simulink model "PMSM_FOC_Average_Inveter"  (R2020b)
settings: Solver=FixedStepAuto  StartTime=0.0  StopTime=10  FixedStep=Fixed_Step_Size  RelTol=1e-3
model workspace (MAT data in the model file):
  wc = Simulink.Parameter
  wc.DataType = 'auto'
  wc.Dimensions = [0 0]
values from neighbouring files (symbols this model uses):
  Angle = 1.0    [Motor_Control_Data.sldd]
  Cosine_table = 1.0 0.99999529 0.99999058 0.99998587 0.99998116 0.99996704 0.99995291 0.99993885 0.99992472 0.99990118 0.99987763 0.99985409 0.9998306 0.99979764 0.99976468 0.99973178 0.99969882 0.99965644 0.99961412 0.99957174 0.99952942 0.99947762 0.99942589 0.99937415 0.99932235 0.9992612 0.99920005 0.99913889 0.99907768 0.99900717 0.99893659 0.99886602 0.99879545 0.99871546 0.99863547 0.99855554 0.99847555 0.    [Motor_Control_Data.sldd]
  Fixed_Step_Size = 1.0E-5    [Motor_Control_Data.sldd]
  Flux = 0.1125    [Motor_Control_Data.sldd]
  ID_Ki = 48.0    [Motor_Control_Data.sldd]
  ID_Kp = 0.84    [Motor_Control_Data.sldd]
  IQ_Ki = 48.0    [Motor_Control_Data.sldd]
  IQ_Kp = 1.869    [Motor_Control_Data.sldd]
  Ld = 0.00014    [Motor_Control_Data.sldd]
  Lq = 0.0003115    [Motor_Control_Data.sldd]
  MTPA_Te_Min = 0.0    [Motor_Control_Data.sldd]
  Pole_Pairs = 4.0    [Motor_Control_Data.sldd]
  PWM_Frequency = 10000.0    [Motor_Control_Data.sldd]
  Sine_table = 0.0 0.0015339879 0.0030679768 0.0046019657 0.0061359555 0.0076698866 0.0092038177 0.010737749 0.012271681 0.013805497 0.015339312 0.016873131 0.018406944 0.019940587 0.021474229 0.023007872 0.024541514 0.026074925 0.027608337 0.029141748 0.03067516 0.032208283 0.033741407 0.035274528 0.036807653 0.038340431 0.039873205 0.04140598 0.042938754 0.04447113 0.046003502 0.047535874 0.049068246 0.0506001    [Motor_Control_Data.sldd]
  Speed_Ki = 10.809    [Motor_Control_Data.sldd]
  Speed_Kp = 0.08    [Motor_Control_Data.sldd]
  Speed_PI_OutputMax = 700.0    [Motor_Control_Data.sldd]
  Speed_PI_OutputMin = -700.0    [Motor_Control_Data.sldd]
  TorqueMode = 0.0    [Motor_Control_Data.sldd]
undefined symbols (not defined in the file or in its folder): Angle_offset, DiscIntNeverNeededParam, FluxWeak_Enable, FluxWeak_Idref_max, FluxWeak_Idref_min, FluxWeak_Ki, FluxWeak_Kp, inverter, MTPA_id_table, MTPA_iq_table, MTPA_Te_Max, Over_modulation, sigbuilder_block, SVPWM
libraries: simulink x7, pid_lib x1, mcbplantlib x1, autolibpmsminterior x1
(part 1 of 2)
settings Model: DataDictionary=Motor_Control_Data.sldd  Creator=jt  LastModifiedBy=Administrator
settings DataIOCC: LimitDataPoints=on  SaveFormat=Array  ReturnWorkspaceOutputs=off
settings OptimizationCC: DefaultParameterBehavior=Inlined  UseDivisionForNetSlopeComputation=on  GainParamInheritBuiltInType=on  UseFloatMulNetSlope=on  InlineInvariantSignals=on  PassReuseOutputArgsAs=Individual arguments  ZeroExternalMemoryAtStartup=off  NoFixptDivByZeroProtection=on  EfficientFloat2IntCast=on  LifeSpan=1  OptimizeBlockOrder=speed  DifferentSizesBufferReuse=on  EfficientTunableParamExpr=on
settings DebuggingCC: AlgebraicLoopMsg=none  MaxConsecutiveZCsMsg=none  SolverPrmCheckMsg=warning  ParameterTunabilityLossMsg=error  AllowSymbolicDim=off  SFUnexpectedBacktrackingDiag=warning  SFNoUnconditionalDefaultTransitionDiag=warning  SFExecutionAtInitializationDiag=none  ArithmeticOperatorsInVariantConditions=warning
settings HardwareCC: ProdBitPerPointer=32  ProdBitPerSizeT=32  ProdBitPerPtrDiffT=32  ProdLargestAtomicInteger=Long  ProdLargestAtomicFloat=Double  ProdEndianess=BigEndian  ProdWordSize=32  ProdLongLongMode=on  ProdHWDeviceType=Freescale->32-bit PowerPC
settings ModelReferenceCC: PropagateSignalLabelsOutOfModel=off
settings SFSimCC: SimUseLocalCustomCode=off  SimParseCustomCode=off  MATLABDynamicMemAlloc=off  CustomCodeUndefinedFunction=UseInterfaceOnly
settings RTWCC: Description=Embedded Coder  SystemTargetFile=ert.tlc  GenCodeOnly=on  TemplateMakefile=ert_default_tmf  GenerateReport=on  RTWUseLocalCustomCode=off  IncludeHyperlinkInReport=on  LaunchReport=on  GenerateTraceInfo=on  GenerateTraceReport=on  GenerateTraceReportSl=on  GenerateTraceReportSf=on  GenerateTraceReportEml=on  GenerateCodeMetricsReport=on
settings CodeAppCC: ForceParamTrailComments=on  IgnoreCustomStorageClasses=off  OperatorAnnotations=on  SimulinkDataObjDesc=on  SFDataObjDesc=on  CustomSymbolStrGlobalVar=rt$N$M  CustomSymbolStrType=$N$M  CustomSymbolStrFcn=$N$M$F  CustomSymbolStrMacro=$N$M  InsertBlockDesc=on
settings ERTTargetCC: GenerateSampleERTMain=on  IncludeMdlTerminateFcn=off  CombineSignalStateStructs=on  SupportAbsoluteTime=off  SupportNonFinite=off  SupportComplex=off  SupportNonInlinedSFcns=on  InlinedParameterPlacement=NonHierarchical  ERTCustomFileTemplate=example_file_process.tlc
settings ConfigComp: CovMetricSettings=dw  CovSaveCumulativeToWorkspaceVar=on  CovSaveSingleToWorkspaceVar=on  CovExternalEMLEnable=off  CovSFcnEnable=off  PSAutoStubLUT=on  DVTestSuiteOptimization=Auto  DVDetectDeadLogic=on  DVDetectActiveLogic=on  DVDetectOutOfBounds=on  DVSaveReport=on  DVDisplayReport=off
settings SimscapeCC: SimscapeNormalizeSystem=off

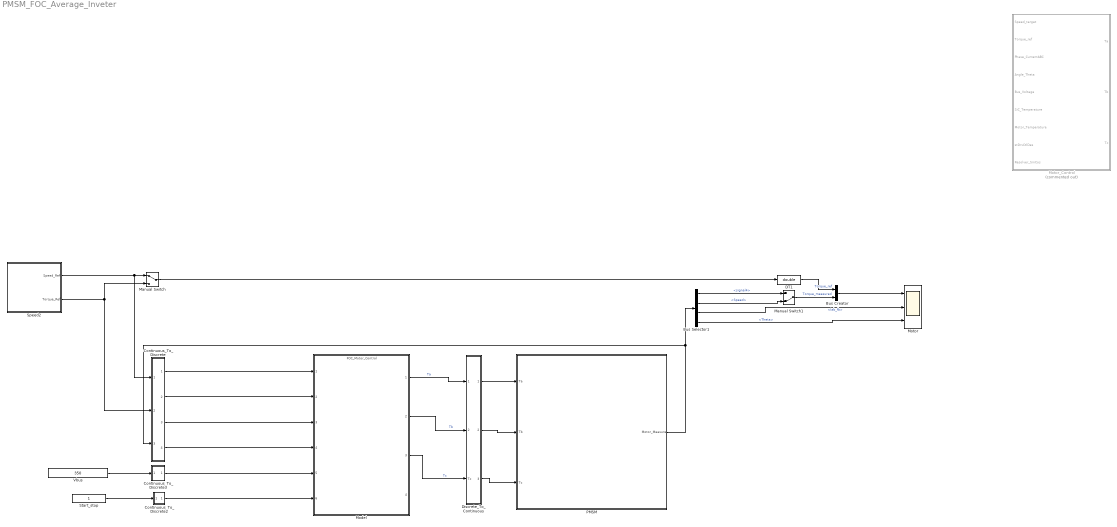
== system PMSM_FOC_Average_Inveter ==
  Bus Creator : BusCreator  Inputs=2
  Bus Selector1 : BusSelector  OutputSignals=signal4,Speed,Iab_fb,Theta
  Continuous_To_Discrete : Subsystem
      mask Display: fprintf('C/D')
  Continuous_To_Discrete2 : Subsystem
      mask Display: fprintf('C/D')
  Continuous_To_Discrete3 : Subsystem
      mask Display: fprintf('C/D')
  DT1 : DataTypeConversion  OutDataTypeStr=double
  Discrete_To_Continuous : Subsystem  Description=""
      mask Display: fprintf('D/C')
  Manual Switch : ManualSwitch
  Manual Switch1 : ManualSwitch  CurrentSetting=0
  Model : ModelReference  ModelNameDialog=FOC_Motor_Control.slx  SimulationMode=Normal  CodeInterface=Top model  ModelReferenceVersion=1.40
  Motor : Scope  NumInputPorts=3
  Motor_Control : Subsystem  Commented=on  TreatAsAtomicUnit=on
  PMSM : Subsystem
      mask Display: image('$imagefile'); % Use "Edit Image" on toolstrip to change.
  Speed2 : Subsystem  Tag=STV Subsys  LoadFcn=sigbuilder_block('load');  StartFcn=sigbuilder_block('start');  StopFcn=sigbuilder_block('stop');  ClipboardFcn=sigbuilder_block('clipboard');  mask(Sigbuilder block){tuvar=[0:10]}
      mask help: Simulink:masks:SigbuilderBlock_MD
      mask init:
      | if ~strcmp(get_param(bdroot(gcbh),'SimulationStatus'),'stopped') tuvar = sigbuilder_block('maskInit'); end
      settings: CopyFcn=sigbuilder_block('copy');  DeleteFcn=sigbuilder_block('delete');  ModelCloseFcn=sigbuilder_block('modelClose');  PreSaveFcn=sigbuilder_block('preSave');  PauseFcn=sigbuilder_block('pause');  ContinueFcn=sigbuilder_block('continue');  NameChangeFcn=sigbuilder_block('namechange');  OpenFcn=sigbuilder_block('open',[48.5 0 906 449 ]);  CloseFcn=sigbuilder_block('close');
      mask Display: plot(0, 0, 100, 100,[2, 2, 32, 32, 2], [68, 8, 8, 68, 68],[32, 2], [38, 38], [32, 19, 2],[53, 60, 44], [32, 17, 17, 2],[16, 16, 31, 31]);txt = getActiveGroup(gcbh);text(2, 100, txt,'verticalAlignment', 'top');
  Start_stop : Constant  OutDataTypeStr=uint8
  Vbus : Constant  Value=350  OutDataTypeStr=single
  wires:
  Discrete_To_Continuous/1(T1) -> PMSM/1(Ta)
  Discrete_To_Continuous/2(T2) -> PMSM/2(Tb)
  Discrete_To_Continuous/3(T3) -> PMSM/3(Tc)
  PMSM/1(Motor_Measure) -> Bus Selector1/1, Continuous_To_Discrete/3(Motor_Measurements)
  Continuous_To_Discrete/4(Theta) -> Model/4
  Model/1 -> Discrete_To_Continuous/1(Ta)  "Ta"
  Model/2 -> Discrete_To_Continuous/2(Tb)  "Tb"
  Model/3 -> Discrete_To_Continuous/3(Tc)  "Tc"
  Bus Creator/1 -> Motor/1
  Bus Selector1/3 -> Motor/2  "<Iab_fb>"
  Speed2/1(Speed_Ref) -> Continuous_To_Discrete/1(Speed_Command), Manual Switch/1
  Continuous_To_Discrete/3(Phase_CurrentABC) -> Model/3
  Bus Selector1/4 -> Motor/3  "<Theta>"
  Start_stop/1 -> Continuous_To_Discrete2/1(Start_stop)
  Speed2/2(Torque_Ref) -> Continuous_To_Discrete/2(Torque_command), Manual Switch/2
  Manual Switch/1 -> DT1/1
  Bus Selector1/1 -> Manual Switch1/1  "<signal4>"
  Bus Selector1/2 -> Manual Switch1/2  "<Speed>"
  Manual Switch1/1 -> Bus Creator/2  "Torque_measured"
  Continuous_To_Discrete2/1(Enable_Disable) -> Model/6
  Continuous_To_Discrete/2(Torque_ref) -> Model/2
  DT1/1 -> Bus Creator/1  "Torque_ref"
  Continuous_To_Discrete/1(Speed_target) -> Model/1
  Vbus/1 -> Continuous_To_Discrete3/1(Bus_Voltage)
  Continuous_To_Discrete3/1(Vbus) -> Model/5

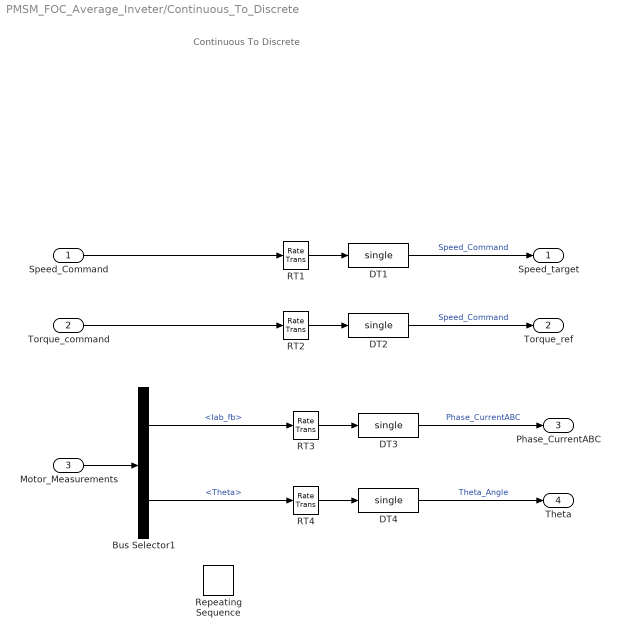
== system PMSM_FOC_Average_Inveter/Continuous_To_Discrete ==
  note: Continuous To Discrete
  Speed_Command : Inport
  Torque_command : Inport  Port=2
  Motor_Measurements : Inport  Port=3
  Bus Selector1 : BusSelector  OutputSignals=Iab_fb,Theta
  DT{1..4} (4 alike) : DataTypeConversion  OutDataTypeStr=single
  RT{1..4} (4 alike) : RateTransition  Integrity=off
  Repeating Sequence : simulink/Sources/Repeating Sequence  rep_seq_t=[0 0.1]  rep_seq_y=[0 6.28]
  Speed_target : Outport
  Torque_ref : Outport  Port=2
  Phase_CurrentABC : Outport  Port=3  PortDimensions=3
  Theta : Outport  Port=4
  wires:
  DT1/1 -> Speed_target/1  "Speed_Command"
  RT1/1 -> DT1/1
  RT3/1 -> DT3/1
  Motor_Measurements/1 -> Bus Selector1/1
  Speed_Command/1 -> RT1/1
  RT4/1 -> DT4/1
  DT4/1 -> Theta/1  "Theta_Angle"
  Bus Selector1/1 -> RT3/1  "<Iab_fb>"
  DT3/1 -> Phase_CurrentABC/1  "Phase_CurrentABC"
  Bus Selector1/2 -> RT4/1  "<Theta>"
  Torque_command/1 -> RT2/1
  RT2/1 -> DT2/1
  DT2/1 -> Torque_ref/1  "Speed_Command"

== system PMSM_FOC_Average_Inveter/Continuous_To_Discrete2 ==
  note: Continuous To Discrete
  Start_stop : Inport
  DT1 : DataTypeConversion  OutDataTypeStr=uint8
  RT1 : RateTransition  Integrity=off
  Enable_Disable : Outport
  wires:
  DT1/1 -> Enable_Disable/1
  RT1/1 -> DT1/1
  Start_stop/1 -> RT1/1

== system PMSM_FOC_Average_Inveter/Continuous_To_Discrete3 ==
  note: Continuous To Discrete
  Bus_Voltage : Inport
  DT2 : DataTypeConversion  OutDataTypeStr=single
  RT2 : RateTransition  Integrity=off
  Vbus : Outport
  wires:
  Bus_Voltage/1 -> RT2/1
  RT2/1 -> DT2/1
  DT2/1 -> Vbus/1

== system PMSM_FOC_Average_Inveter/Discrete_To_Continuous ==
  note: Discrete To Continuous
  Ta : Inport
  Tb : Inport  Port=2
  Tc : Inport  Port=3
  DT : DataTypeConversion
  DT1 : DataTypeConversion
  DT2 : DataTypeConversion
  RT : RateTransition  Integrity=off
  RT1 : RateTransition  Integrity=off
  RT2 : RateTransition  Integrity=off
  T1 : Outport
  T2 : Outport  Port=2
  T3 : Outport  Port=3
  wires:
  DT/1 -> RT/1
  Ta/1 -> DT/1  "Tabc"
  DT1/1 -> RT1/1
  Tb/1 -> DT1/1  "Tabc"
  DT2/1 -> RT2/1
  Tc/1 -> DT2/1  "Tabc"
  RT/1 -> T1/1  "Tabc"
  RT1/1 -> T2/1  "Tabc"
  RT2/1 -> T3/1  "Tabc"

== system PMSM_FOC_Average_Inveter/Motor_Control ==
  Speed_target : Inport
  Torque_ref : Inport  Port=2  OutMin=0  OutMax=2*pi
  Phase_CurrentABC : Inport  Port=3  PortDimensions=3
  Angle_Theta : Inport  Port=4  OutMin=0  OutMax=2*pi
  Bus_Voltage : Inport  Port=5
  SiC_Temperature : Inport  Port=6
  Motor_Temperature : Inport  Port=7
  stDrvCtlDes : Inport  Port=8
  Resolver_SinCos : Inport  Port=9  OutMin=0  OutMax=2*pi
  Motor_Control_Function : Subsystem
  Ta : Outport
  Tb : Outport  Port=2
  Tc : Outport  Port=3
  wires:
  Motor_Control_Function/2(Tb) -> Tb/1
  Motor_Control_Function/3(Tc) -> Tc/1
  Motor_Control_Function/1(Ta) -> Ta/1
  Speed_target/1 -> Motor_Control_Function/1(Speed_target)  "Speed_target"
  Phase_CurrentABC/1 -> Motor_Control_Function/2(Phase_CurrentABC)  "Phase_CurrentABC"
  Angle_Theta/1 -> Motor_Control_Function/3(Angle_Theta)  "Angle_Theta"
  Resolver_SinCos/1 -> Motor_Control_Function/4(Resolver_SinCos)  "Resolver_signal"
  stDrvCtlDes/1 -> Motor_Control_Function/16(stDrvCtlDes)
  Bus_Voltage/1 -> Motor_Control_Function/5(Bus_voltage)
  SiC_Temperature/1 -> Motor_Control_Function/6(SiC_Temperature)
  Motor_Temperature/1 -> Motor_Control_Function/7(Motor_Temperature)
  Torque_ref/1 -> Motor_Control_Function/22(Torque_ref)

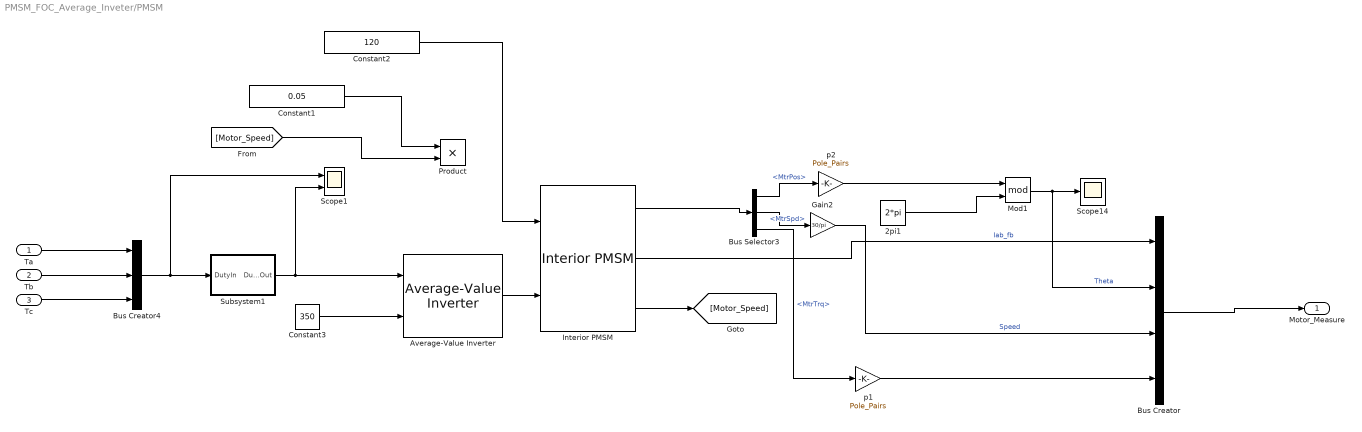
== system PMSM_FOC_Average_Inveter/PMSM ==
  Ta : Inport
  Tb : Inport  Port=2
  Tc : Inport  Port=3
  2pi1 : Constant  Value=2*pi
  Average-Value Inverter : mcbplantlib/Average-Value Inverter
  Bus Creator : BusCreator  Inputs=4
  Bus Creator4 : BusCreator  Inputs=3
  Bus Selector3 : BusSelector  OutputSignals=MtrPos,MtrSpd,MtrTrq
  Constant1 : Constant  Value=0.05
  Constant2 : Constant  Value=120
  Constant3 : Constant  Value=350
  Gain2 : Gain  Gain=30/pi  OutDataTypeStr=Inherit: Same as input  ParamDataTypeStr=Inherit: Same as input
  Interior PMSM : autolibpmsminterior/Interior PMSM  port_config=Torque  sim_type=Discrete  Ts=Fixed_Step_Size  P=Pole_Pairs  Rs=R  Ldq=[Ld Lq]  KConstText=Permanent flux linkage constant (lambda_pm):  lambda_pm=Flux  Ke=159.9771  mechanical=[0.002,0,0]  idq0=[0 0]  theta_init=0  omega_init=0  KConst=Flux  lambda_pm_calc=Flux  Kt=0.07  RefBlkName='autolibpmsminterior/Interior PMSM'  aMode=5
      settings: SourceProductBaseCode=PW,MT,UV,VE,VP
  Mod1 : Math  Operator=mod  SaturateOnIntegerOverflow=on
  Product : Product
  Scope1 : Scope  NumInputPorts=2
  Scope14 : Scope
  Subsystem1 : Subsystem
  p1 : Gain  Gain=Pole_Pairs  OutDataTypeStr=Inherit: Same as input  ParamDataTypeStr=Inherit: Same as input
  p2 : Gain  Gain=Pole_Pairs  OutDataTypeStr=Inherit: Same as input  ParamDataTypeStr=Inherit: Same as input
  Motor_Measure : Outport
  wires:
  Mod1/1 -> Bus Creator/2, Scope14/1  "Theta"
  Bus Creator/1 -> Motor_Measure/1
  Tc/1 -> Bus Creator4/3
  Interior PMSM/1 -> Bus Selector3/1
  Average-Value Inverter/1 -> Interior PMSM/2
  Subsystem1/1(DutyOut) -> Scope1/2, Average-Value Inverter/1
  Constant3/1 -> Average-Value Inverter/2
  Interior PMSM/2 -> Bus Creator/1  "Iab_fb"
  Bus Creator4/1 -> Subsystem1/1(DutyIn), Scope1/1
  Bus Selector3/2 -> Gain2/1  "<MtrSpd>"
  Bus Selector3/1 -> p2/1  "<MtrPos>"
  p2/1 -> Mod1/1
  2pi1/1 -> Mod1/2
  Gain2/1 -> Bus Creator/3  "Speed"
  Ta/1 -> Bus Creator4/1
  Tb/1 -> Bus Creator4/2
  Interior PMSM/3 -> [Motor_Speed]
  Bus Selector3/3 -> p1/1  "<MtrTrq>"
  p1/1 -> Bus Creator/4
  [Motor_Speed] -> Product/2
  Constant1/1 -> Product/1
  Constant2/1 -> Interior PMSM/1

== system PMSM_FOC_Average_Inveter/Speed2 ==
  Demux : Demux  Tag=STV Demux  Outputs=2
      settings: DisplayOption=none
  FromWs : FromWorkspace  Tag=STV FromWs  VariableName=tuvar
      SigBuilderData=|
      | common.afterFinalStr = 'Extrapolate'
      | common.sampleTime = 0
      | dataSet.timeRange = [0 10]
      | dataSet.name = 'Target Speed'
      | sbobj.Groups.Name = 'Target Speed'
      | sbobj.Groups.Signals(1).Name = 'Speed_Ref'
      | sbobj.Groups.Signals(1).XData = [0 4.51 10]
      | sbobj.Groups.Signals(1).YData = [2000 2000 2000]
      | sbobj.Groups.Signals(2).Name = 'Torque_Ref'
      | sbobj.Groups.Signals(2).XData = [0 1.26 1.26 2.9 5.44 5.44 7.94 10]
      | sbobj.Groups.Signals(2).YData = [170 170 169.5 170.5 170.5 170 170 170]
  Speed_Ref : Outport  Tag=STV Outport
  Torque_Ref : Outport  Tag=STV Outport  Port=2
  wires:
  FromWs/1 -> Demux/1
  Demux/1 -> Speed_Ref/1
  Demux/2 -> Torque_Ref/1

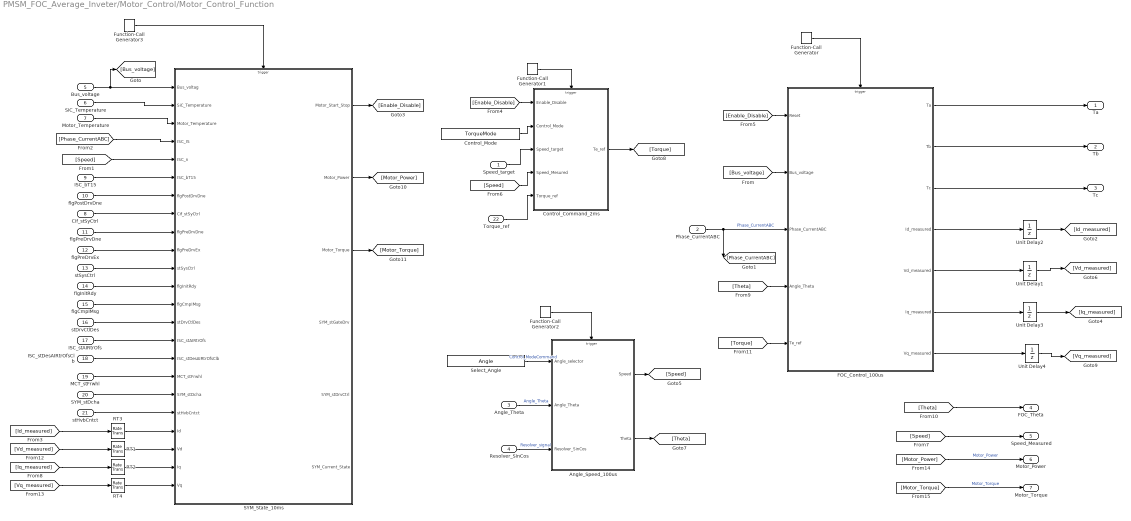
== system PMSM_FOC_Average_Inveter/Motor_Control/Motor_Control_Function ==
  Speed_target : Inport
  Phase_CurrentABC : Inport  Port=2  PortDimensions=3
  Angle_Theta : Inport  Port=3  OutMin=0  OutMax=2*pi
  Resolver_SinCos : Inport  Port=4  OutMin=0  OutMax=2*pi
  Bus_voltage : Inport  Port=5
  SiC_Temperature : Inport  Port=6
  Motor_Temperature : Inport  Port=7
  Cif_stSyCtrl : Inport  Port=8
  ISC_bT15 : Inport  Port=9
  flgPostDrvDne : Inport  Port=10
  flgPreDrvDne : Inport  Port=11
  flgPreDrvEx : Inport  Port=12
  stSysCtrl : Inport  Port=13
  flgInitRdy : Inport  Port=14
  flgCmpIMsg : Inport  Port=15
  stDrvCtlDes : Inport  Port=16
  ISC_stAIRtrOfs : Inport  Port=17
  "ISC_stDesAIRtrOfsClb " : Inport  Port=18
  MCT_stFrwhl : Inport  Port=19
  SYM_stDcha : Inport  Port=20
  stHvbCntct : Inport  Port=21
  Torque_ref : Inport  Port=22  OutMin=0  OutMax=2*pi
  Angle_Speed_100us : Subsystem
      settings: RTWSystemCode=Nonreusable function  RTWFcnNameOpts=Use subsystem name  RTWFileNameOpts=Use subsystem name
  Control_Command_2ms : Subsystem  TreatAsAtomicUnit=on
      settings: RTWSystemCode=Nonreusable function  RTWFcnNameOpts=Use subsystem name  RTWFileNameOpts=Use subsystem name  FunctionInterfaceSpec=Allow arguments (Optimized)
  Control_Mode : Constant  Value=TorqueMode
  FOC_Control_100us : Subsystem  TreatAsAtomicUnit=on
      settings: RTWSystemCode=Nonreusable function  RTWFcnNameOpts=Use subsystem name  RTWFileNameOpts=Use subsystem name  FunctionInterfaceSpec=Allow arguments (Optimized)
  Function-Call Generator : simulink/Ports & Subsystems/Function-Call Generator  sample_time=Task_100us  numberOfIterations=1  DisallowWideOutput=off
  Function-Call Generator1 : simulink/Ports & Subsystems/Function-Call Generator  sample_time=Task_2ms  numberOfIterations=1  DisallowWideOutput=off
  Function-Call Generator2 : simulink/Ports & Subsystems/Function-Call Generator  sample_time=Task_100us  numberOfIterations=1  DisallowWideOutput=off
  Function-Call Generator3 : simulink/Ports & Subsystems/Function-Call Generator  sample_time=Task_10ms  numberOfIterations=1  DisallowWideOutput=off
  RT{1..4} (4 alike) : RateTransition  Integrity=off
  SYM_State_10ms : Subsystem
      settings: RTWSystemCode=Nonreusable function  RTWFcnNameOpts=Use subsystem name  RTWFileNameOpts=Use subsystem name
  Select_Angle : Constant  Value=Angle
  Unit Delay{1..4} (4 alike) : UnitDelay  SampleTime=-1  HasFrameUpgradeWarning=on
  Ta : Outport
  Tb : Outport  Port=2
  Tc : Outport  Port=3
  FOC_Theta : Outport  Port=4
  Speed_Measured : Outport  Port=5
  Motor_Power : Outport  Port=6
  Motor_Torque : Outport  Port=7
  wires:
  Resolver_SinCos/1 -> Angle_Speed_100us/3(Resolver_SinCos)  "Resolver_signal"
  Function-Call Generator1/1 -> Control_Command_2ms/Trigger
  Control_Mode/1 -> Control_Command_2ms/2(Control_Mode)
  Angle_Theta/1 -> Angle_Speed_100us/2(Angle_Theta)  "Angle_Theta"
  Function-Call Generator/1 -> FOC_Control_100us/Trigger
  Phase_CurrentABC/1 -> [Phase_CurrentABC], FOC_Control_100us/3(Phase_CurrentABC)  "Phase_CurrentABC"
  FOC_Control_100us/3(Tc) -> Tc/1
  Select_Angle/1 -> Angle_Speed_100us/1(Angle_selector)  "Control_ModeCommand"
  Speed_target/1 -> Control_Command_2ms/3(Speed_target)
  FOC_Control_100us/2(Tb) -> Tb/1
  FOC_Control_100us/1(Ta) -> Ta/1
  Function-Call Generator2/1 -> Angle_Speed_100us/Trigger
  Function-Call Generator3/1 -> SYM_State_10ms/Trigger
  SYM_State_10ms/1(Motor_Start_Stop) -> [Enable_Disable]
  [Enable_Disable] -> Control_Command_2ms/1(Enable_Disable)
  [Enable_Disable] -> FOC_Control_100us/1(Reset)
  Angle_Speed_100us/1(Speed) -> [Speed]
  [Speed] -> Control_Command_2ms/4(Speed_Mesured)
  [Speed] -> Speed_Measured/1
  Angle_Speed_100us/2(Theta) -> [Theta]
  [Theta] -> FOC_Control_100us/4(Angle_Theta)
  [Theta] -> FOC_Theta/1
  Control_Command_2ms/1(Te_ref) -> [Torque]
  [Torque] -> FOC_Control_100us/5(Te_ref)
  Cif_stSyCtrl/1 -> SYM_State_10ms/8(Cif_stSyCtrl)
  ISC_bT15/1 -> SYM_State_10ms/6(ISC_bT15)
  flgPostDrvDne/1 -> SYM_State_10ms/7(flgPostDrvDne)
  flgPreDrvDne/1 -> SYM_State_10ms/9(flgPreDrvDne)
  flgPreDrvEx/1 -> SYM_State_10ms/10(flgPreDrvEx)
  stSysCtrl/1 -> SYM_State_10ms/11(stSysCtrl)
  flgInitRdy/1 -> SYM_State_10ms/12(flgInitRdy)
  flgCmpIMsg/1 -> SYM_State_10ms/13(flgCmpIMsg)
  stDrvCtlDes/1 -> SYM_State_10ms/14(stDrvCtlDes)
  ISC_stAIRtrOfs/1 -> SYM_State_10ms/15(ISC_stAIRtrOfs)
  "ISC_stDesAIRtrOfsClb "/1 -> SYM_State_10ms/16("ISC_stDesAIRtrOfsClb ")
  MCT_stFrwhl/1 -> SYM_State_10ms/17(MCT_stFrwhl)
  SYM_stDcha/1 -> SYM_State_10ms/18(SYM_stDcha)
  stHvbCntct/1 -> SYM_State_10ms/19(stHvbCntct)
  Bus_voltage/1 -> [Bus_voltage], SYM_State_10ms/1(Bus_voltag)
  SiC_Temperature/1 -> SYM_State_10ms/2(SiC_Temperature)
  Motor_Temperature/1 -> SYM_State_10ms/3(Motor_Temperature)
  [Speed] -> SYM_State_10ms/5(ISC_n)
  [Phase_CurrentABC] -> SYM_State_10ms/4(ISC_IS)
  FOC_Control_100us/6(Iq_measured) -> Unit Delay3/1
  FOC_Control_100us/7(Vq_measured) -> Unit Delay4/1
  FOC_Control_100us/4(Id_measured) -> Unit Delay2/1
  FOC_Control_100us/5(Vd_measured) -> Unit Delay1/1
  Unit Delay2/1 -> [Id_measured]
  Unit Delay1/1 -> [Vd_measured]
  Unit Delay3/1 -> [Iq_measured]
  Unit Delay4/1 -> [Vq_measured]
  [Iq_measured] -> RT2/1
  [Id_measured] -> RT3/1
  [Vd_measured] -> RT1/1
  [Vq_measured] -> RT4/1
  SYM_State_10ms/2(Motor_Power) -> [Motor_Power]
  [Motor_Power] -> Motor_Power/1  "Motor_Power"
  RT3/1 -> SYM_State_10ms/20(Id)
  RT1/1 -> SYM_State_10ms/21(Vd)
  RT2/1 -> SYM_State_10ms/22(Iq)
  RT4/1 -> SYM_State_10ms/23(Vq)
  [Bus_voltage] -> FOC_Control_100us/2(Bus_voltage)
  SYM_State_10ms/3(Motor_Torque) -> [Motor_Torque]
  [Motor_Torque] -> Motor_Torque/1  "Motor_Torque"
  Torque_ref/1 -> Control_Command_2ms/5(Torque_ref)

== system PMSM_FOC_Average_Inveter/PMSM/Subsystem1 ==
  DutyIn : Inport
  Constant : Constant  Value=0.5  SampleTime=-1
  Gain : Gain  Gain=1/9999  ParamDataTypeStr=single
  Gain1 : Gain  Gain=-1
  Sum : Sum  Inputs=|+-
  Sum1 : Sum  Inputs=|++
  DutyOut : Outport
  wires:
  Sum/1 -> Gain1/1
  Constant/1 -> Sum1/2, Sum/2
  DutyIn/1 -> Gain/1
  Gain1/1 -> Sum1/1
  Gain/1 -> Sum/1
  Sum1/1 -> DutyOut/1

== system PMSM_FOC_Average_Inveter/Motor_Control/Motor_Control_Function/Angle_Speed_100us ==
  Angle_selector : Inport
  Angle_Theta : Inport  Port=2  OutMin=0  OutMax=2*pi
  Resolver_SinCos : Inport  Port=3  OutMin=0  OutMax=2*pi
  Trigger : TriggerPort  TriggerType=function-call  VariantControl=Variant  SampleTimeType=periodic  SampleTime=-1  PortDimensions=1
  Merge : Merge
  Merge1 : Merge
  Resolver_Observer : Subsystem
      settings: RTWSystemCode=Nonreusable function  RTWFcnNameOpts=Use subsystem name
  Speed_Resolver : Subsystem  TreatAsAtomicUnit=on
      settings: RTWSystemCode=Nonreusable function  RTWFcnNameOpts=Use subsystem name
  Switch Case : SwitchCase  CaseConditions={1,2}
  Speed : Outport
  Theta : Outport  Port=2
  wires:
  Resolver_SinCos/1 -> Resolver_Observer/1(Resolver_SinCos)  "Resolver_signal"
  [Observer_Angle] -> Resolver_Observer/Action
  Resolver_Observer/2(Obser_Theta) -> Merge1/1
  Merge/1 -> Speed/1
  Merge1/1 -> Theta/1
  Angle_selector/1 -> Switch Case/1  "Control_ModeCommand"
  Switch Case/3 -> [default]
  Switch Case/1 -> [Atan_Angle]
  Switch Case/2 -> [Observer_Angle]
  Speed_Resolver/1(Speed_out) -> Merge/1
  Angle_Theta/1 -> Speed_Resolver/1(Theta)  "Angle_Theta"
  [Atan_Angle] -> Speed_Resolver/Action
  Resolver_Observer/1(Obser_Speed) -> Merge/2
  Speed_Resolver/2(Dir_Angle) -> Merge1/2

== system PMSM_FOC_Average_Inveter/Motor_Control/Motor_Control_Function/Control_Command_2ms ==
  Enable_Disable : Inport
  Control_Mode : Inport  Port=2
  Speed_target : Inport  Port=3
  Speed_Mesured : Inport  Port=4  OutMin=0  OutMax=2*pi
  Torque_ref : Inport  Port=5  OutMin=0  OutMax=2*pi
  Trigger : TriggerPort  TriggerType=function-call  VariantControl=Variant  SampleTimeType=periodic  SampleTime=-1  PortDimensions=1
  Control_Command_2ms : Subsystem  TreatAsAtomicUnit=on
      settings: RTWSystemCode=Nonreusable function  RTWFcnNameOpts=Use subsystem name  RTWFileNameOpts=Use subsystem name  FunctionInterfaceSpec=Allow arguments (Optimized)
  Te_ref : Outport
  wires:
  Control_Mode/1 -> Control_Command_2ms/2(Control_Mode)
  Speed_target/1 -> Control_Command_2ms/3(Speed_target)
  Speed_Mesured/1 -> Control_Command_2ms/4(Speed_Mesured)  "Speed_Measured"
  Control_Command_2ms/1(Te_ref) -> Te_ref/1
  Enable_Disable/1 -> Control_Command_2ms/1(Reset)
  Torque_ref/1 -> Control_Command_2ms/5(Torque_ref)

== system PMSM_FOC_Average_Inveter/Motor_Control/Motor_Control_Function/FOC_Control_100us ==
  Reset : Inport
  Bus_voltage : Inport  Port=2
  Phase_CurrentABC : Inport  Port=3  PortDimensions=3
  Angle_Theta : Inport  Port=4  OutMin=0  OutMax=2*pi
  Te_ref : Inport  Port=5
  Trigger : TriggerPort  TriggerType=function-call  VariantControl=Variant  SampleTimeType=periodic  SampleTime=-1  PortDimensions=1
  FOC : Subsystem  TreatAsAtomicUnit=on
      settings: RTWSystemCode=Nonreusable function  RTWFcnNameOpts=Use subsystem name
  MTPA : Subsystem  TreatAsAtomicUnit=on
      settings: RTWSystemCode=Nonreusable function  RTWFcnNameOpts=Use subsystem name
  Ta : Outport
  Tb : Outport  Port=2
  Tc : Outport  Port=3
  Id_measured : Outport  Port=4
  Vd_measured : Outport  Port=5
  Iq_measured : Outport  Port=6
  Vq_measured : Outport  Port=7
  wires:
  FOC/1(Ta) -> Ta/1  "Ta"
  FOC/2(Tb) -> Tb/1  "Tb"
  FOC/3(Tc) -> Tc/1  "Tc"
  Angle_Theta/1 -> FOC/5(Angle_Theta)  "Angle_Theta"
  Phase_CurrentABC/1 -> FOC/6(Phase_CurrentABC)  "Phase_CurrentABC"
  MTPA/1(Id_ref) -> FOC/3(Id_target)
  MTPA/2(Iq_ref) -> FOC/4(Iq_target)
  Te_ref/1 -> MTPA/1(Te_ref)
  Reset/1 -> FOC/1(Reset)
  FOC/6(Iq_measured) -> Iq_measured/1
  FOC/7(Vq_measured) -> Vq_measured/1
  FOC/4(Id_measured) -> Id_measured/1
  FOC/5(Vd_measured) -> Vd_measured/1
  Bus_voltage/1 -> FOC/2(Bus_voltage)

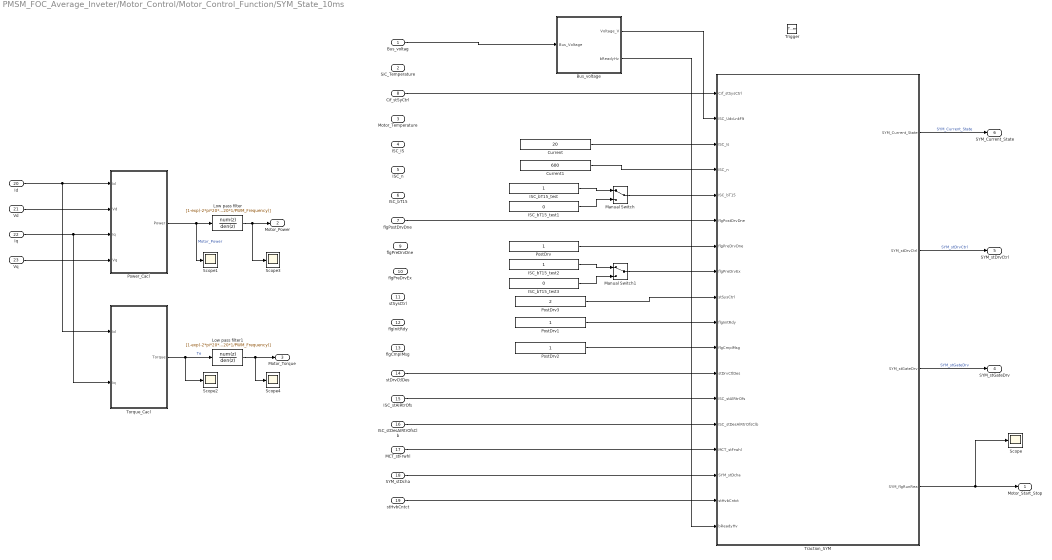
== system PMSM_FOC_Average_Inveter/Motor_Control/Motor_Control_Function/SYM_State_10ms ==
  Bus_voltag : Inport
  SiC_Temperature : Inport  Port=2
  Motor_Temperature : Inport  Port=3
  ISC_IS : Inport  Port=4
  ISC_n : Inport  Port=5
  ISC_bT15 : Inport  Port=6
  flgPostDrvDne : Inport  Port=7
  Cif_stSyCtrl : Inport  Port=8
  flgPreDrvDne : Inport  Port=9
  flgPreDrvEx : Inport  Port=10
  stSysCtrl : Inport  Port=11
  flgInitRdy : Inport  Port=12
  flgCmpIMsg : Inport  Port=13
  stDrvCtlDes : Inport  Port=14
  ISC_stAIRtrOfs : Inport  Port=15
  "ISC_stDesAIRtrOfsClb " : Inport  Port=16
  MCT_stFrwhl : Inport  Port=17
  SYM_stDcha : Inport  Port=18
  stHvbCntct : Inport  Port=19
  Id : Inport  Port=20
  Vd : Inport  Port=21
  Iq : Inport  Port=22
  Vq : Inport  Port=23
  Trigger : TriggerPort  TriggerType=function-call  VariantControl=Variant  SampleTimeType=periodic  SampleTime=-1  PortDimensions=1
  Bus_voltage : Subsystem
  Current : Constant  Value=20  OutDataTypeStr=int16
  Current1 : Constant  Value=600  OutDataTypeStr=int16
  ISC_bT15_test : Constant  OutDataTypeStr=boolean
  ISC_bT15_test1 : Constant  Value=0  OutDataTypeStr=boolean
  ISC_bT15_test2 : Constant  OutDataTypeStr=uint8
  ISC_bT15_test3 : Constant  Value=0  OutDataTypeStr=uint8
  Low pass filter : DiscreteTransferFcn  Numerator=[1-exp(-2*pi*20*1/PWM_Frequency)]  Denominator=[1 -exp(-2*pi*20*1/PWM_Frequency)]
  Low pass filter1 : DiscreteTransferFcn  Numerator=[1-exp(-2*pi*20*1/PWM_Frequency)]  Denominator=[1 -exp(-2*pi*20*1/PWM_Frequency)]
  Manual Switch : ManualSwitch
  Manual Switch1 : ManualSwitch
  PostDrv : Constant  OutDataTypeStr=uint8
  PostDrv1 : Constant  OutDataTypeStr=boolean
  PostDrv2 : Constant  OutDataTypeStr=uint8
  PostDrv3 : Constant  Value=2  OutDataTypeStr=uint8
  Power_Cacl : Subsystem
  Scope{,1..4} (5 alike) : Scope
  Torque_Cacl : Subsystem
  Traction_SYM : Stateflow chart  TreatAsAtomicUnit=on
  Motor_Start_Stop : Outport
  Motor_Power : Outport  Port=2
  Motor_Torque : Outport  Port=3
  SYM_stGateDrv : Outport  Port=4
  SYM_stDrvCtrl : Outport  Port=5
  SYM_Current_State : Outport  Port=6
  wires:
  Cif_stSyCtrl/1 -> Traction_SYM/1(Cif_stSysCtrl)
  PostDrv/1 -> Traction_SYM/7(flgPreDrvDne)
  flgPostDrvDne/1 -> Traction_SYM/6(flgPostDrvDne)
  PostDrv1/1 -> Traction_SYM/10(flgInitRdy)
  PostDrv2/1 -> Traction_SYM/11(flgCmpIMsg)
  Bus_voltag/1 -> Bus_voltage/1(Bus_Voltage)
  Bus_voltage/1(Voltage_V) -> Traction_SYM/2(ISC_UdcLnkFlt)
  Bus_voltage/2(bReadyHv) -> Traction_SYM/18(bReadyHv)
  ISC_bT15_test/1 -> Manual Switch/1
  ISC_bT15_test1/1 -> Manual Switch/2
  Manual Switch/1 -> Traction_SYM/5(ISC_bT15)
  Manual Switch1/1 -> Traction_SYM/8(flgPreDrvEx)
  ISC_bT15_test2/1 -> Manual Switch1/1
  ISC_bT15_test3/1 -> Manual Switch1/2
  Current/1 -> Traction_SYM/3(ISC_Is)
  Current1/1 -> Traction_SYM/4(ISC_n)
  PostDrv3/1 -> Traction_SYM/9(stSysCtrl)
  Traction_SYM/4(SYM_flgRunRea) -> Motor_Start_Stop/1, Scope/1
  stDrvCtlDes/1 -> Traction_SYM/12(stDrvCtlDes)
  ISC_stAIRtrOfs/1 -> Traction_SYM/13(ISC_stAlRtrOfs)
  "ISC_stDesAIRtrOfsClb "/1 -> Traction_SYM/14(ISC_stDesAlRtrOfsClb)
  MCT_stFrwhl/1 -> Traction_SYM/15(MCT_stFrwhl)
  SYM_stDcha/1 -> Traction_SYM/16(SYM_stDcha)
  stHvbCntct/1 -> Traction_SYM/17(stHvbCntct)
  Iq/1 -> Torque_Cacl/2(Iq), Power_Cacl/3(Iq)
  Vq/1 -> Power_Cacl/4(Vq)
  Power_Cacl/1(Power) -> Scope1/1, Low pass filter/1  "Motor_Power"
  Vd/1 -> Power_Cacl/2(Vd)
  Id/1 -> Torque_Cacl/1(Id), Power_Cacl/1(Id)
  Low pass filter/1 -> Scope3/1, Motor_Power/1
  Torque_Cacl/1(Torque) -> Low pass filter1/1, Scope2/1  "Te"
  Low pass filter1/1 -> Motor_Torque/1, Scope4/1
  Traction_SYM/3(SYM_stGateDrv) -> SYM_stGateDrv/1  "SYM_stGateDrv"
  Traction_SYM/2(SYM_stDrvCtrl) -> SYM_stDrvCtrl/1  "SYM_stDrvCtrl"
  Traction_SYM/1(SYM_Current_State) -> SYM_Current_State/1  "SYM_Current_State"

== system PMSM_FOC_Average_Inveter/Motor_Control/Motor_Control_Function/Angle_Speed_100us/Resolver_Observer ==
  Resolver_SinCos : Inport
  Action Port : ActionPort
  Angle_calibration : Subsystem  TreatAsAtomicUnit=on
      settings: RTWSystemCode=Nonreusable function  RTWFcnNameOpts=Use subsystem name
  Resolver_Angle_cacl : Subsystem  TreatAsAtomicUnit=on
      settings: RTWSystemCode=Nonreusable function  RTWFcnNameOpts=Use subsystem name  RTWFileNameOpts=Use subsystem name  FunctionInterfaceSpec=Allow arguments (Optimized)
  Scope : Scope
  Scope1 : Scope
  Obser_Speed : Outport
  Obser_Theta : Outport  Port=2
  wires:
  Resolver_Angle_cacl/1(Velocity) -> Scope/1, Obser_Speed/1  "Obser_Speed"
  Resolver_Angle_cacl/2(Angle) -> Angle_calibration/1(Angle_input)
  Resolver_SinCos/1 -> Resolver_Angle_cacl/1(Sin_Cos)
  Angle_calibration/1(Angle_output) -> Scope1/1, Obser_Theta/1  "Obser_Angle"

== system PMSM_FOC_Average_Inveter/Motor_Control/Motor_Control_Function/Angle_Speed_100us/Speed_Resolver ==
  Theta : Inport
  Action Port : ActionPort
  DT2 : DataTypeConversion  OutDataTypeStr=single
  Speed_cacl : Subsystem  TreatAsAtomicUnit=on
      settings: RTWSystemCode=Nonreusable function  RTWFcnNameOpts=Use subsystem name
  Speed_out : Outport
  Dir_Angle : Outport  Port=2
  wires:
  Theta/1 -> DT2/1, Speed_cacl/1(position)
  Speed_cacl/1(Speed_RPM) -> Speed_out/1  "Speed_RPM_Filtered"
  DT2/1 -> Dir_Angle/1  "Direct_Angle"

== system PMSM_FOC_Average_Inveter/Motor_Control/Motor_Control_Function/Control_Command_2ms/Control_Command_2ms ==
  Reset : Inport
  Control_Mode : Inport  Port=2
  Speed_target : Inport  Port=3
  Speed_Mesured : Inport  Port=4  OutMin=0  OutMax=2*pi
  Torque_ref : Inport  Port=5  OutMin=0  OutMax=2*pi
  Merge : Merge
  Speed_PI : Subsystem  TreatAsAtomicUnit=on  SystemSampleTime=inverter.Ts
      settings: RTWSystemCode=Nonreusable function
  Switch Case : SwitchCase  CaseConditions={0,1}
  Switch Case Action Subsystem : Subsystem  TreatAsAtomicUnit=on
      settings: RTWSystemCode=Nonreusable function
  Te_ref : Outport
  wires:
  Switch Case Action Subsystem/1(Iq_out) -> Merge/2
  Torque_ref/1 -> Switch Case Action Subsystem/1(Iq_in)
  Switch Case/3 -> [default]
  [Torque_Mode] -> Switch Case Action Subsystem/Action
  Switch Case/2 -> [Torque_Mode]
  Switch Case/1 -> [Speed_Mode]
  Control_Mode/1 -> Switch Case/1
  [Speed_Mode] -> Speed_PI/Action
  Speed_PI/1(Iq_ref) -> Merge/1  "Iq_ref"
  Merge/1 -> Te_ref/1
  Speed_target/1 -> Speed_PI/1(Speed_Command)
  Speed_Mesured/1 -> Speed_PI/2(Speed_Measured)  "Speed_Mesured"
  Reset/1 -> Speed_PI/3(Reset)

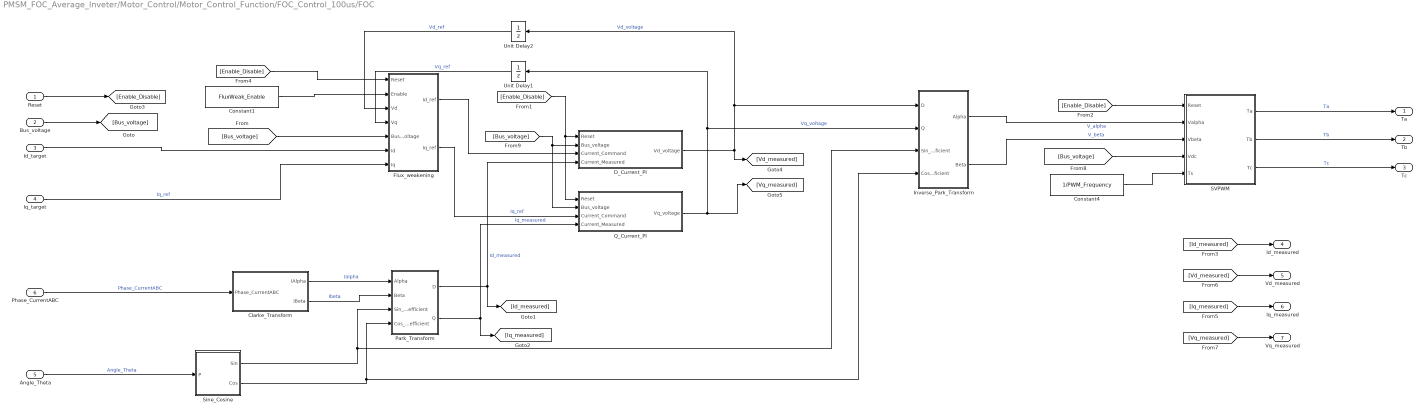
== system PMSM_FOC_Average_Inveter/Motor_Control/Motor_Control_Function/FOC_Control_100us/FOC ==
  Reset : Inport
  Bus_voltage : Inport  Port=2
  Id_target : Inport  Port=3
  Iq_target : Inport  Port=4
  Angle_Theta : Inport  Port=5  OutMin=0  OutMax=2*pi
  Phase_CurrentABC : Inport  Port=6  PortDimensions=3
  Clarke_Transform : Subsystem  TreatAsAtomicUnit=on
      settings: RTWSystemCode=Nonreusable function  RTWFcnNameOpts=Use subsystem name
  Constant1 : Constant  Value=FluxWeak_Enable  OutDataTypeStr=single
  Constant4 : Constant  Value=1/PWM_Frequency  OutDataTypeStr=single
  D_Current_PI : Subsystem  TreatAsAtomicUnit=on
      settings: RTWSystemCode=Nonreusable function  RTWFcnNameOpts=Use subsystem name
  "Flux_weakening " : Subsystem
  Inverse_Park_Transform : Subsystem  TreatAsAtomicUnit=on
      settings: RTWSystemCode=Nonreusable function  RTWFcnNameOpts=Use subsystem name
      mask Display:
      | port_label('input',1,'D')
      | port_label('input',2,'Q')
      | port_label('input',3,'Sin')
      | port_label('input',4,'Cos')
      | port_label('output',1,'\alpha','texmode', 'on')
      | port_label('output',2,'\beta','texmode', 'on')
  Park_Transform : Subsystem  TreatAsAtomicUnit=on
      settings: RTWSystemCode=Nonreusable function  RTWFcnNameOpts=Use subsystem name
      mask Display:
      | port_label('input',1,'\alpha','texmode', 'on')
      | port_label('input',2,'\beta','texmode', 'on')
      | port_label('input',3,'Sin')
      | port_label('input',4,'Cos')
      | port_label('output',1,'D')
      | port_label('output',2,'Q')
  Q_Current_PI : Subsystem  TreatAsAtomicUnit=on
      settings: RTWSystemCode=Nonreusable function  RTWFcnNameOpts=Use subsystem name
  SVPWM : Subsystem  AncestorBlock=SVPWM/SVPWM  TreatAsAtomicUnit=on  RTWFcnName=SVPWM  RTWFileName=SVPWM
      settings: RTWSystemCode=Nonreusable function  RTWFcnNameOpts=Use subsystem name
      mask Display:
      | plot([0.000 0.020 0.041 0.061 0.082 0.102 0.122 0.143 0.163 0.184 0.204 0.224 0.245 0.265 0.286 0.306 0.327 0.347 0.367 0.388 0.408 0.429 0.449 0.469 0.490 0.510 0.531 0.551 0.571 0.592 0.612 0.633 0.653 0.673 0.694 0.714 0.735 0.755 0.776 0.796 0.816 0.837 0.857 0.878 0.898 0.918 0.939 0.959 0.980 1.000 ], ...
      |      [0.500 0.586 0.671 0.753 0.831 0.858 0.875 0.885 0.890 0.887 0.879 0.864 0.844 0.855 0.872 0.884 0.889 0.888 0.881 0.867 0.847 0.793 0.713 0.629 0.543 0.457 0.371 0.287 0.207 0.153 0.133 0.119 0.112 0.111 0.116 0.128 0.145 0.156 0.136 0.121 0.113 0.110 0.115 0.125 0.142 0.169 0.247 0.329 0.414 0.500 ])
  Sine_Cosine : Subsystem  TreatAsAtomicUnit=on
      settings: RTWSystemCode=Nonreusable function  RTWFcnNameOpts=Use subsystem name
  Unit Delay1 : UnitDelay  SampleTime=-1  HasFrameUpgradeWarning=on
  Unit Delay2 : UnitDelay  SampleTime=-1  HasFrameUpgradeWarning=on
  Ta : Outport
  Tb : Outport  Port=2
  Tc : Outport  Port=3
  Id_measured : Outport  Port=4
  Vd_measured : Outport  Port=5
  Iq_measured : Outport  Port=6
  Vq_measured : Outport  Port=7
  wires:
  Park_Transform/1(D) -> D_Current_PI/4(Current_Measured), [Id_measured]  "Id_measured"
  Constant4/1 -> SVPWM/5(Ts)
  SVPWM/3(Tc) -> Tc/1  "Tc"
  SVPWM/2(Tb) -> Tb/1  "Tb"
  Park_Transform/2(Q) -> Q_Current_PI/4(Current_Measured), [Iq_measured]  "Iq_measured"
  Sine_Cosine/2(Cos) -> Park_Transform/4(Cos_Coefficient), Inverse_Park_Transform/4(Cos_Coefficient)
  Sine_Cosine/1(Sin) -> Park_Transform/3(Sin_Coefficient), Inverse_Park_Transform/3(Sin_Coefficient)
  [Bus_voltage] -> SVPWM/4(Vdc)
  D_Current_PI/1(Vd_voltage) -> Unit Delay2/1, Inverse_Park_Transform/1(D), [Vd_measured]  "Vd_voltage"
  Q_Current_PI/1(Vq_voltage) -> [Vq_measured], Unit Delay1/1, Inverse_Park_Transform/2(Q)  "Vq_voltage"
  SVPWM/1(Ta) -> Ta/1  "Ta"
  Id_target/1 -> "Flux_weakening "/6(Id)
  Iq_target/1 -> "Flux_weakening "/7(Iq)  "Iq_ref"
  Clarke_Transform/2(IBeta) -> Park_Transform/2(Beta)  "Ibeta"
  Clarke_Transform/1(IAlpha) -> Park_Transform/1(Alpha)  "Ialpha"
  Unit Delay2/1 -> "Flux_weakening "/3(Vd)  "Vd_ref"
  Unit Delay1/1 -> "Flux_weakening "/4(Vq)  "Vq_ref"
  "Flux_weakening "/2(Iq_ref) -> Q_Current_PI/3(Current_Command)  "Iq_ref"
  Constant1/1 -> "Flux_weakening "/2(Enable)
  Inverse_Park_Transform/1(Alpha) -> SVPWM/2(Valpha)  "V_alpha"
  Inverse_Park_Transform/2(Beta) -> SVPWM/3(Vbeta)  "V_beta"
  Phase_CurrentABC/1 -> Clarke_Transform/1(Phase_CurrentABC)  "Phase_CurrentABC"
  Angle_Theta/1 -> Sine_Cosine/1(P)  "Angle_Theta"
  "Flux_weakening "/1(Id_ref) -> D_Current_PI/3(Current_Command)
  Reset/1 -> [Enable_Disable]
  [Enable_Disable] -> "Flux_weakening "/1(Reset)
  [Enable_Disable] -> Q_Current_PI/1(Reset), D_Current_PI/1(Reset)
  [Enable_Disable] -> SVPWM/1(Reset)
  [Iq_measured] -> Iq_measured/1
  [Id_measured] -> Id_measured/1
  [Vd_measured] -> Vd_measured/1
  [Vq_measured] -> Vq_measured/1
  Bus_voltage/1 -> [Bus_voltage]
  [Bus_voltage] -> "Flux_weakening "/5(Bus_voltage)
  [Bus_voltage] -> Q_Current_PI/2(Bus_voltage), D_Current_PI/2(Bus_voltage)

== system PMSM_FOC_Average_Inveter/Motor_Control/Motor_Control_Function/FOC_Control_100us/MTPA ==
  Te_ref : Inport
  1-D Lookup Table4 : Lookup_n-D  NumberOfTableDimensions=1  LookupTableObject=''  BreakpointsForDimension1=single(linspace(MTPA_Te_Min,MTPA_Te_Max,length(MTPA_id_table)));  BreakpointsForDimension1FirstPoint=10  BreakpointsForDimension2FirstPoint=10  BreakpointsForDimension1Spacing=12  BreakpointsForDimension2Spacing=12  IndexSearchMethod=Evenly spaced points  Table=MTPA_id_table  InterpMethod=Flat  DiagnosticForOutOfRangeInput=Error  InternalRulePriority=Speed  RndMeth=Simplest  InputSameDT=on
  1-D Lookup Table5 : Lookup_n-D  NumberOfTableDimensions=1  LookupTableObject=''  BreakpointsForDimension1=single(linspace(MTPA_Te_Min,MTPA_Te_Max,length(MTPA_id_table)));  BreakpointsForDimension1FirstPoint=10  BreakpointsForDimension2FirstPoint=10  BreakpointsForDimension1Spacing=12  BreakpointsForDimension2Spacing=12  IndexSearchMethod=Evenly spaced points  Table=MTPA_iq_table  InterpMethod=Flat  DiagnosticForOutOfRangeInput=Error  InternalRulePriority=Speed  RndMeth=Simplest  InputSameDT=on
  Saturation : Saturate  UpperLimit=MTPA_Te_Max-0.01  LowerLimit=MTPA_Te_Min+0.01
  Saturation1 : Saturate  UpperLimit=MTPA_Te_Max-0.01  LowerLimit=MTPA_Te_Min+0.01
  Id_ref : Outport
  Iq_ref : Outport  Port=2
  wires:
  Te_ref/1 -> Saturation1/1, Saturation/1
  Saturation/1 -> 1-D Lookup Table4/1
  Saturation1/1 -> 1-D Lookup Table5/1
  1-D Lookup Table4/1 -> Id_ref/1
  1-D Lookup Table5/1 -> Iq_ref/1

== system PMSM_FOC_Average_Inveter/Motor_Control/Motor_Control_Function/SYM_State_10ms/Bus_voltage ==
  Bus_Voltage : Inport
  ISC_bT15_test : Constant  Value=300  OutDataTypeStr=int16
  If1 : If  IfExpression=u1>450  ElseIfExpressions=u1<20
  Merge : Merge  Inputs=3
  Normal_Voltage : Subsystem  TreatAsAtomicUnit=on
      settings: RTWSystemCode=Nonreusable function  RTWFcnNameOpts=Use subsystem name
  Over_Voltage : Subsystem  TreatAsAtomicUnit=on
      settings: RTWSystemCode=Nonreusable function  RTWFcnNameOpts=Use subsystem name
  Under_Voltage : Subsystem  TreatAsAtomicUnit=on
      settings: RTWSystemCode=Nonreusable function  RTWFcnNameOpts=Use subsystem name
  Voltage_V : Outport
  bReadyHv : Outport  Port=2
  wires:
  ISC_bT15_test/1 -> Voltage_V/1, If1/1
  If1/1 -> Over_Voltage/Action
  Merge/1 -> bReadyHv/1
  Over_Voltage/1(Over_voltage) -> Merge/1
  If1/2 -> Under_Voltage/Action
  If1/3 -> Normal_Voltage/Action
  Under_Voltage/1(Under_voltage) -> Merge/2
  Normal_Voltage/1(Normal_Voltage) -> Merge/3

== system PMSM_FOC_Average_Inveter/Motor_Control/Motor_Control_Function/SYM_State_10ms/Power_Cacl ==
  Id : Inport
  Vd : Inport  Port=2
  Iq : Inport  Port=3
  Vq : Inport  Port=4
  Add : Sum
  Product : Product
  Product1 : Product
  Power : Outport
  wires:
  Id/1 -> Product/1
  Vd/1 -> Product/2
  Iq/1 -> Product1/1
  Vq/1 -> Product1/2
  Product/1 -> Add/1
  Product1/1 -> Add/2
  Add/1 -> Power/1

== system PMSM_FOC_Average_Inveter/Motor_Control/Motor_Control_Function/SYM_State_10ms/Torque_Cacl ==
  Id : Inport
  Iq : Inport  Port=2
  Constant : Constant  Value=3/2  OutDataTypeStr=single
  Constant1 : Constant  Value=Pole_Pairs  OutDataTypeStr=single
  Constant2 : Constant  Value=Flux  OutDataTypeStr=single
  Constant3 : Constant  Value=Ld  OutDataTypeStr=single
  Constant4 : Constant  Value=Lq  OutDataTypeStr=single
  Product{,1..4} (5 alike) : Product
  Subtract : Sum
  Subtract1 : Sum  Inputs=+-
  Torque : Outport
  wires:
  Constant1/1 -> Product/1
  Constant/1 -> Product/2
  Constant2/1 -> Product1/1
  Iq/1 -> Product1/2, Product3/1
  Product1/1 -> Subtract/1
  Constant3/1 -> Subtract1/1
  Constant4/1 -> Subtract1/2
  Subtract1/1 -> Product2/1
  Id/1 -> Product2/2
  Product2/1 -> Product3/2
  Product3/1 -> Subtract/2
  Product/1 -> Product4/1
  Subtract/1 -> Product4/2
  Product4/1 -> Torque/1

== system PMSM_FOC_Average_Inveter/Motor_Control/Motor_Control_Function/Angle_Speed_100us/Resolver_Observer/Angle_calibration ==
  Angle_input : Inport
  Angle_offset : Constant  Value=Angle_offset
  If Action Subsystem1 : Subsystem  TreatAsAtomicUnit=on
  If Action Subsystem2 : Subsystem  TreatAsAtomicUnit=on
  If1 : If  IfExpression=u1 > 6.283185307
  Merge1 : Merge
  Subtract1 : Sum
  Angle_output : Outport
  wires:
  Angle_input/1 -> Subtract1/1
  Merge1/1 -> Angle_output/1
  Angle_offset/1 -> Subtract1/2  "Control_ModeCommand"
  If1/1 -> If Action Subsystem2/Action
  If1/2 -> If Action Subsystem1/Action
  If Action Subsystem2/1(Out1) -> Merge1/1
  Subtract1/1 -> If Action Subsystem1/1(In1), If Action Subsystem2/1(In1), If1/1
  If Action Subsystem1/1(Out1) -> Merge1/2

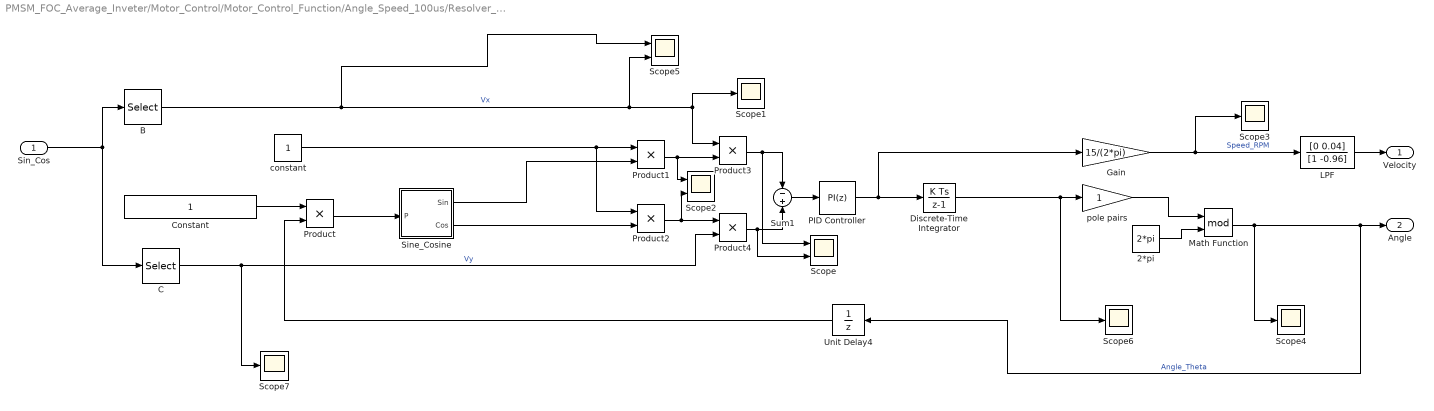
== system PMSM_FOC_Average_Inveter/Motor_Control/Motor_Control_Function/Angle_Speed_100us/Resolver_Observer/Resolver_Angle_cacl ==
  Sin_Cos : Inport
  2*pi : Constant  Value=2*pi  OutDataTypeStr=single  SampleTime=-1
  B : Selector  IndexMode=Zero-based  InputPortWidth=2  IndexOptions=Index vector (dialog)  Indices=0  OutputSizes=1
  C : Selector  IndexMode=Zero-based  InputPortWidth=2  IndexOptions=Index vector (dialog)  Indices=1  OutputSizes=1
  Constant : Constant  OutDataTypeStr=single  SampleTime=-1
  Discrete-Time Integrator : DiscreteIntegrator  SampleTime=-1  ICPrevOutput=DiscIntNeverNeededParam  ICPrevScaledInput=DiscIntNeverNeededParam
  Gain : Gain  Gain=15/(2*pi)
  LPF : DiscreteFilter  Numerator=[0 0.04]  Denominator=[1 -0.96]
  Math Function : Math  Operator=mod  SignedPower=on  SaturateOnIntegerOverflow=on
  PID Controller : pid_lib/PID Controller  Controller=PI  Form=Parallel  TimeDomain=Discrete-time  UseExternalTs=off  SampleTime=-1  IntegratorMethod=Forward Euler  FilterMethod=Forward Euler  ControllerParametersSource=internal  P=141  I=10000  D=0  UseFilter=off  N=100  TunerSelectOption=Transfer Function Based (PID Tuner App)  InitialConditionSource=internal  InitialConditionForIntegrator=0  InitialConditionForFilter=0  DifferentiatorICPrevScaledInput=0  ExternalReset=none  TrackingMode=off  Kt=1  LimitOutput=off  SatLimitsSource=internal  UpperSaturationLimit=inf  LowerSaturationLimit=-inf  LinearizeAsGain=on  AntiWindupMode=none  Kb=1  POutMin=[]  POutMax=[]  IOutMin=[]  IOutMax=[]  DOutMin=[]  DOutMax=[]  NOutMin=[]  NOutMax=[]  SumOutMin=[]  SumOutMax=[]  SaturationOutMin=[]  SaturationOutMax=[]  PParamMin=[]  PParamMax=[]  IParamMin=[]  IParamMax=[]  DParamMin=[]  DParamMax=[]  NParamMin=[]  NParamMax=[]  KbParamMin=[]  KbParamMax=[]  KtParamMin=[]  KtParamMax=[]  KbOutMin=[]  KbOutMax=[]  KtOutMin=[]  KtOutMax=[]  IntegratorOutMin=[]  IntegratorOutMax=[]  FilterOutMin=[]  FilterOutMax=[]  SumI1OutMin=[]  SumI1OutMax=[]  SumI2OutMin=[]  SumI2OutMax=[]  SumI3OutMin=[]  SumI3OutMax=[]  SumI4OutMin=[]  SumI4OutMax=[]  SumDOutMin=[]  SumDOutMax=[]  DifferentiatorOutMin=[]  DifferentiatorOutMax=[]  FilterDiffOutCoefMin=[]  FilterDiffOutCoefMax=[]  ReciprocalOutMin=[]  ReciprocalOutMax=[]  SumDenOutMin=[]  SumDenOutMax=[]  SumNumOutMin=[]  SumNumOutMax=[]  DivideOutMin=[]  DivideOutMax=[]  UdiffTsProdOutMin=[]  UdiffTsProdOutMax=[]  NTsProdOutMin=[]  NTsProdOutMax=[]  UintegralTsProdOutMin=[]  UintegralTsProdOutMax=[]  UngainTsProdOutMin=[]  UngainTsProdOutMax=[]  IntegratorContinuousStateAttributes=''  IntegratorStateMustResolveToSignalObject=off  IntegratorRTWStateStorageClass=Auto  FilterContinuousStateAttributes=''  FilterStateMustResolveToSignalObject=off  FilterRTWStateStorageClass=Auto  ParallelPVariant=InternalParameters  IdealPVariant=Disabled  IVariant=InternalParameters  DVariant=Disabled  IntegratorVariant=Discrete  SatVariant=Disabled  AWVariant=Passthrough  PCopyVariant=Disabled  TRVariant=Disabled  FdbkBlocksVariant=Forward  IdealPFdbkVariant=Disabled  SatFdbkVariant=Disabled  DerivativeFilterVariant=Disabled  NVariant=Disabled  NCopyVariant=Disabled_SignalSpec  FilterICVariant=Disabled  IntegratorICVariant=InternalICs  ExternalResetVariant=Disabled  TRSumVariant=Passthrough  SumFdbkVariant=Disabled  SumVariant=Sum_PI  TsampFilterVariant=InternalTs  TsampNgainVariant=Passthrough  TsampIntegralVariant=Passthrough  ExternalSaturationOutDataTypeStr=Inherit: Same as second input
  Product : Product  OutDataTypeStr=single
  Product{1..4} (4 alike) : Product
  Scope : Scope  NumInputPorts=2
  Scope{1,3..4,6..7} (5 alike) : Scope
  Scope2 : Scope  NumInputPorts=2
  Scope5 : Scope  NumInputPorts=2
  Sine_Cosine : Subsystem  TreatAsAtomicUnit=on
      settings: RTWSystemCode=Nonreusable function  RTWFcnNameOpts=Use subsystem name
  Sum1 : Sum  Inputs=-+
  Unit Delay4 : UnitDelay  SampleTime=-1  HasFrameUpgradeWarning=on
  constant : Constant  OutDataTypeStr=single
  "pole pairs " : Gain  OutDataTypeStr=single
  Velocity : Outport  VectorParamsAs1DForOutWhenUnconnected=off
  Angle : Outport  Port=2  VectorParamsAs1DForOutWhenUnconnected=off
  wires:
  Product2/1 -> Scope2/2, Product4/1
  Product4/1 -> Scope/2, Sum1/2
  Sin_Cos/1 -> C/1, B/1
  Unit Delay4/1 -> Product/2
  Sum1/1 -> PID Controller/1
  Product3/1 -> Scope/1, Sum1/1
  Constant/1 -> Product/1
  constant/1 -> Product2/1, Product1/1
  Product/1 -> Sine_Cosine/1(P)
  Sine_Cosine/1(Sin) -> Product1/2
  Product1/1 -> Scope2/1, Product3/2
  Math Function/1 -> Unit Delay4/1, Angle/1, Scope4/1  "Angle_Theta"
  Gain/1 -> LPF/1, Scope3/1  "Speed_RPM"
  Discrete-Time Integrator/1 -> Scope6/1, "pole pairs "/1
  "pole pairs "/1 -> Math Function/1
  PID Controller/1 -> Discrete-Time Integrator/1, Gain/1
  2*pi/1 -> Math Function/2
  B/1 -> Scope1/1, Product3/1, Scope5/2, Scope5/1  "Vx"
  C/1 -> Product4/2, Scope7/1  "Vy"
  LPF/1 -> Velocity/1
  Sine_Cosine/2(Cos) -> Product2/2

== system PMSM_FOC_Average_Inveter/Motor_Control/Motor_Control_Function/Angle_Speed_100us/Speed_Resolver/Speed_cacl ==
  position : Inport  OutMin=-4*pi  OutMax=4*pi
      settings: AttributesFormatString="------------------\\nMin =  %<OutMin>\\nMax =  %<OutMax>"
  Constant : Constant  Value=pi/(2^31 -1)/(1/PWM_Frequency)  OutDataTypeStr=single
  Constant1 : Constant  Value=1/Pole_Pairs  OutDataTypeStr=single
  Difference_Wrap : Sum  Inputs=+-  AccumDataTypeStr=int32  OutDataTypeStr=int32
  Difference_to_Single : DataTypeConversion  OutDataTypeStr=single
  Gain : Gain  Gain=60/(2*pi)
  LPF : DiscreteFilter  Numerator=[0 0.5]  Denominator=[1 -0.5]
  Position_Delay : Delay  DelayLength=1
  Product : Product
  Product1 : Product
  Scale_Input : Gain  Gain=((2^31) - 1)/(4*pi)  ParamDataTypeStr=single  OutDataTypeStr=single
      settings: AttributesFormatString=---------------------------------\n%<Gain>
  Wrap_To_Pi : Gain  Gain=4  RndMeth=Simplest  OutDataTypeStr=Inherit: Same as input  ParamDataTypeStr=Inherit: Same as input
  Speed_RPM : Outport  VectorParamsAs1DForOutWhenUnconnected=off
  wires:
  position/1 -> Scale_Input/1  "position"
  Difference_to_Single/1 -> Product/2
  Wrap_To_Pi/1 -> Difference_Wrap/1, Position_Delay/1
  Position_Delay/1 -> Difference_Wrap/2
  Scale_Input/1 -> Wrap_To_Pi/1
  Difference_Wrap/1 -> Difference_to_Single/1
  Product1/1 -> LPF/1
  LPF/1 -> Speed_RPM/1  "Speed_measured"
  Constant/1 -> Product/1
  Constant1/1 -> Product1/1
  Product/1 -> Gain/1  "We"
  Gain/1 -> Product1/2

== system PMSM_FOC_Average_Inveter/Motor_Control/Motor_Control_Function/Control_Command_2ms/Control_Command_2ms/Speed_PI ==
  Speed_Command : Inport
  Speed_Measured : Inport  Port=2
  Reset : Inport  Port=3
  Action Port : ActionPort
  Add2 : Sum  Inputs=|+-
  Speed_PI : Subsystem
  Iq_ref : Outport  VectorParamsAs1DForOutWhenUnconnected=off
  wires:
  Speed_Command/1 -> Add2/1
  Speed_Measured/1 -> Add2/2
  Add2/1 -> Speed_PI/1(PI_input)  "currentControlError"
  Speed_PI/1(PI_out) -> Iq_ref/1
  Reset/1 -> Speed_PI/2(Reset)

== system PMSM_FOC_Average_Inveter/Motor_Control/Motor_Control_Function/Control_Command_2ms/Control_Command_2ms/Switch Case Action Subsystem ==
  Iq_in : Inport
  Action Port : ActionPort
  Iq_out : Outport
  wires:
  Iq_in/1 -> Iq_out/1

== system PMSM_FOC_Average_Inveter/Motor_Control/Motor_Control_Function/FOC_Control_100us/FOC/Clarke_Transform ==
  Phase_CurrentABC : Inport  PortDimensions=3
  Clark1 : Subsystem  TreatAsAtomicUnit=on
  Scope : Scope  NumInputPorts=2
  IAlpha : Outport  VectorParamsAs1DForOutWhenUnconnected=off
  IBeta : Outport  Port=2  VectorParamsAs1DForOutWhenUnconnected=off
  wires:
  Clark1/1(Ialpha) -> IAlpha/1, Scope/1
  Clark1/2(Ibeta) -> IBeta/1, Scope/2
  Phase_CurrentABC/1 -> Clark1/1(Iabc)

== system PMSM_FOC_Average_Inveter/Motor_Control/Motor_Control_Function/FOC_Control_100us/FOC/D_Current_PI ==
  Reset : Inport
  Bus_voltage : Inport  Port=2
  Current_Command : Inport  Port=3
  Current_Measured : Inport  Port=4
  Add2 : Sum  Inputs=|+-
  ID_Control : Subsystem
  Vd_voltage : Outport  VectorParamsAs1DForOutWhenUnconnected=off
  wires:
  Current_Command/1 -> Add2/1
  Current_Measured/1 -> Add2/2
  Add2/1 -> ID_Control/3(Err)  "currentControlError"
  ID_Control/1(PI_Out) -> Vd_voltage/1
  Reset/1 -> ID_Control/1(Reset)
  Bus_voltage/1 -> ID_Control/2(Bus_voltage)

== system PMSM_FOC_Average_Inveter/Motor_Control/Motor_Control_Function/FOC_Control_100us/FOC/Flux_weakening  ==
  Reset : Inport
  Enable : Inport  Port=2
  Vd : Inport  Port=3
  Vq : Inport  Port=4
  Bus_voltage : Inport  Port=5
  Id : Inport  Port=6
  Iq : Inport  Port=7
  If1 : If  IfExpression=u1 ==1
  Merge : Merge
  Merge1 : Merge
  Subsystem : Subsystem
  Subsystem1 : Subsystem
  Id_ref : Outport
  Iq_ref : Outport  Port=2
  wires:
  Enable/1 -> If1/1
  If1/1 -> Subsystem/Action
  If1/2 -> Subsystem1/Action
  Id/1 -> Subsystem/4(Id), Subsystem1/1(Id)
  Iq/1 -> Subsystem/5(Iq), Subsystem1/2(Iq)
  Vd/1 -> Subsystem/2(Vd)
  Vq/1 -> Subsystem/3(Vq)
  Subsystem/1(Id_ref) -> Merge/1
  Subsystem1/1(Id_ref) -> Merge/2
  Subsystem/2(Iq_ref) -> Merge1/1
  Subsystem1/2(Iq_ref) -> Merge1/2
  Merge1/1 -> Iq_ref/1
  Merge/1 -> Id_ref/1
  Reset/1 -> Subsystem/1(Reset)
  Bus_voltage/1 -> Subsystem/6(Bus_voltage)
